simulink model "lab02_fechado"  (Simulink 10.3)
settings: Solver=VariableStepAuto  StartTime=0.0  StopTime=10.0  RelTol=1e-3
values from neighbouring files (symbols this model uses):
  c_1 = 0.2254    [lab02.mat]    (also in lab03.mat; lab04.mat; lab05.mat; lab06.mat)
  c_r = 0.0144    [lab02.mat]    (also in lab03.mat; lab04.mat; lab05.mat; lab06.mat)
  Denth = [1 1.28221624265 36.6770172992 23.5454339835 -528.584013296]    [lab03.mat]    (also in lab04.mat; lab05.mat; lab06.mat; lab07.mat)
  Denx = [1 1.28221624265 36.6770172992 23.5454339835 -528.584013296]    [lab03.mat]    (also in lab04.mat; lab05.mat; lab06.mat; lab07.mat)
  g = 9.8    [lab02.mat]    (also in lab03.mat; lab04.mat; lab05.mat; lab06.mat)
  Ja = 0.06904489    [lab02.mat]    (also in lab03.mat; lab04.mat; lab05.mat = 0.06191089; lab06.mat = 0.06932089)
  Jb = 0.04317025    [lab02.mat]    (also in lab03.mat; lab04.mat; lab05.mat = 0.03603625; lab06.mat = 0.04344625)
  k_a = 2546    [lab02.mat]    (also in lab03.mat; lab04.mat; lab05.mat; lab06.mat)
  k_f = 0.0013    [lab02.mat]    (also in lab03.mat; lab04.mat; lab05.mat; lab06.mat)
  k_hw = 2088.32    [lab02.mat]    (also in lab03.mat; lab04.mat; lab05.mat; lab06.mat)
  k_p = 2    [lab02.mat]    (also in lab03.mat = 0.256097247605; lab04.mat = 0.137612608424; lab05.mat = 0.280842058008; lab06.mat = 0.012)
  k_pf = 1    [lab02.mat]    (also in lab03.mat; lab04.mat; lab05.mat; lab06.mat)
  k_s = 32    [lab02.mat]    (also in lab03.mat; lab04.mat; lab05.mat; lab06.mat)
  k_v = 0.01    [lab02.mat]    (also in lab03.mat; lab04.mat; lab05.mat; lab06.mat)
  k_x = 50200    [lab02.mat]    (also in lab03.mat; lab04.mat; lab05.mat; lab06.mat)
  l_0 = 0.33    [lab02.mat]    (also in lab03.mat; lab04.mat; lab05.mat; lab06.mat)
  l_c = -0.0458067226891    [lab03.mat]    (also in lab04.mat; lab05.mat = -0.0295602240896; lab06.mat = -0.0463669467787; lab07.mat = -0.0295602240896)
  m_1 = 0.2376    [lab02.mat]    (also in lab03.mat; lab04.mat; lab05.mat; lab06.mat)
  m_2 = 1.785    [lab02.mat]    (also in lab03.mat; lab04.mat; lab05.mat; lab06.mat)
  Numth = [0 0 -7.64415309154 -7.25165028128 227.008182718]    [lab03.mat]    (also in lab04.mat; lab05.mat; lab06.mat; lab07.mat)
  Numx = [0 0 6.73132472896 2.24532116671 3.20735046038]    [lab03.mat]    (also in lab04.mat; lab05.mat; lab06.mat; lab07.mat)
settings Model: Creator=kisdev  LastModifiedBy=kisdev
settings SolverCC: AlgebraicLoopSolver=Auto
settings DataIOCC: SaveFormat=Dataset  SignalLoggingSaveFormat=Dataset  ReturnWorkspaceOutputs=on
settings OptimizationCC: ExpressionDepthLimit=128  LifeSpan=auto
settings DebuggingCC: UnderspecifiedInitializationDetection=Simplified  MergeDetectMultiDrivingBlocksExec=error  FcnCallInpInsideContextMsg=error  StateNameClashWarn=none  SFUnexpectedBacktrackingDiag=error  SFNoUnconditionalDefaultTransitionDiag=error  SFExecutionAtInitializationDiag=warning  SFMachineParentedDataDiag=error  ArithmeticOperatorsInVariantConditions=error
settings HardwareCC: ProdBitPerPointer=64  ProdBitPerSizeT=64  ProdBitPerPtrDiffT=64  ProdLargestAtomicFloat=Float  ProdIntDivRoundTo=Zero  ProdEndianess=LittleEndian  ProdWordSize=64  ProdHWDeviceType=Intel->x86-64 (Windows64)
settings ModelReferenceCC: PropagateSignalLabelsOutOfModel=on
settings SFSimCC: SimUseLocalCustomCode=on  CustomCodeUndefinedFunction=FilterOut
settings RTWCC: RTWUseLocalCustomCode=on
settings CodeAppCC: StateflowObjectComments=off
settings GRTTargetCC: TargetLangStandard=C99 (ISO)  CombineOutputUpdateFcns=on  GRTInterface=off
settings ConfigComp: CovMetricSettings=dwe  CovSaveCumulativeToWorkspaceVar=off  CovSaveSingleToWorkspaceVar=off  CovExternalEMLEnable=on

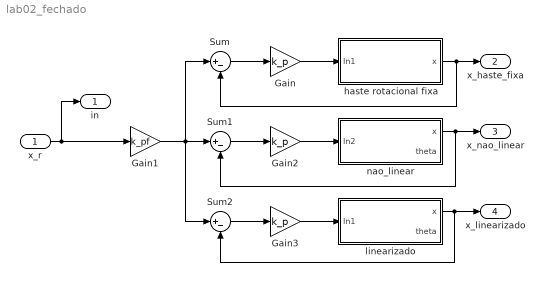
== system lab02_fechado ==
  x_r : Inport
  Gain : Gain  Gain=k_p
  Gain1 : Gain  Gain=k_pf
  Gain2 : Gain  Gain=k_p
  Gain3 : Gain  Gain=k_p
  Sum : Sum  Inputs=|+-
  Sum1 : Sum  Inputs=|+-
  Sum2 : Sum  Inputs=|+-
  haste rotacional fixa : Subsystem
  linearizado : Subsystem
  nao_linear : Subsystem
  in : Outport
  x_haste_fixa : Outport  Port=2
  x_nao_linear : Outport  Port=3
  x_linearizado : Outport  Port=4
  wires:
  x_r/1 -> in/1, Gain1/1
  Gain1/1 -> Sum2/1, Sum1/1, Sum/1
  Sum/1 -> Gain/1
  Sum1/1 -> Gain2/1
  Sum2/1 -> Gain3/1
  nao_linear/1(x) -> Sum1/2, x_nao_linear/1
  Gain2/1 -> nao_linear/1(In2)
  Gain/1 -> haste rotacional fixa/1(In1)
  haste rotacional fixa/1(x) -> Sum/2, x_haste_fixa/1
  Gain3/1 -> linearizado/1(In1)
  linearizado/1(x) -> Sum2/2, x_linearizado/1

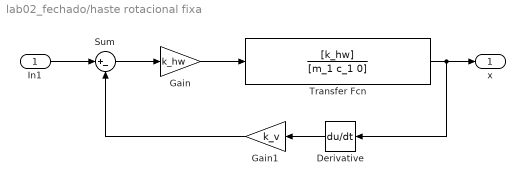
== system lab02_fechado/haste rotacional fixa ==
  In1 : Inport
  Derivative : Derivative
  Gain : Gain  Gain=k_hw
  Gain1 : Gain  Gain=k_v
  Sum : Sum  Inputs=|+-
  Transfer Fcn : TransferFcn  Numerator=[k_hw]  Denominator=[m_1 c_1 0]
  x : Outport
  wires:
  Transfer Fcn/1 -> Derivative/1, x/1
  Derivative/1 -> Gain1/1
  Gain1/1 -> Sum/2
  Gain/1 -> Transfer Fcn/1
  In1/1 -> Sum/1
  Sum/1 -> Gain/1

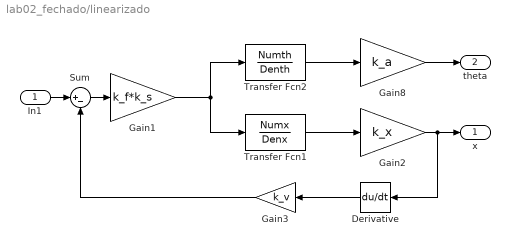
== system lab02_fechado/linearizado ==
  In1 : Inport
  Derivative : Derivative
  Gain1 : Gain  Gain=k_f*k_s
  Gain2 : Gain  Gain=k_x
  Gain3 : Gain  Gain=k_v
  Gain8 : Gain  Gain=k_a
  Sum : Sum  Inputs=|+-
  Transfer Fcn1 : TransferFcn  Numerator=Numx  Denominator=Denx
  Transfer Fcn2 : TransferFcn  Numerator=Numth  Denominator=Denth
  x : Outport
  theta : Outport  Port=2
  wires:
  Sum/1 -> Gain1/1
  In1/1 -> Sum/1
  Gain2/1 -> x/1, Derivative/1
  Transfer Fcn2/1 -> Gain8/1
  Gain1/1 -> Transfer Fcn1/1, Transfer Fcn2/1
  Transfer Fcn1/1 -> Gain2/1
  Gain8/1 -> theta/1
  Gain3/1 -> Sum/2
  Derivative/1 -> Gain3/1

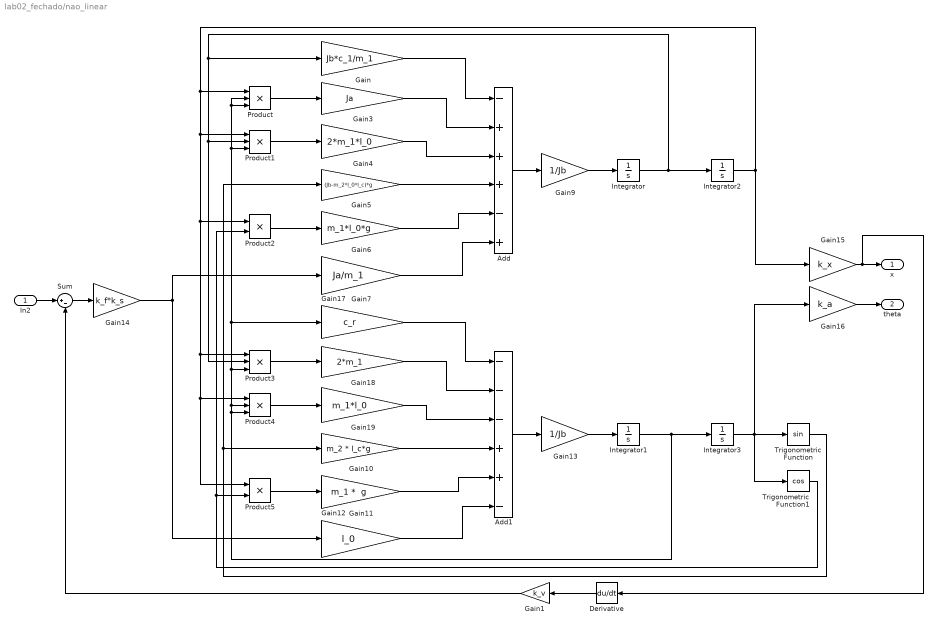
== system lab02_fechado/nao_linear ==
  In2 : Inport
  Add : Sum  Inputs=-+++-+
  Add1 : Sum  Inputs=---++-
  Derivative : Derivative
  Gain : Gain  Gain=Jb*c_1/m_1
  Gain1 : Gain  Gain=k_v
  Gain10 : Gain  Gain=m_2 * l_c*g
  Gain11 : Gain  Gain="m_1 *  g"
  Gain12 : Gain  Gain=l_0
  Gain13 : Gain  Gain=1/Jb
  Gain14 : Gain  Gain=k_f*k_s
  Gain15 : Gain  Gain=k_x
  Gain16 : Gain  Gain=k_a
  Gain17 : Gain  Gain=c_r
  Gain18 : Gain  Gain=2*m_1
  Gain19 : Gain  Gain=m_1*l_0
  Gain3 : Gain  Gain=Ja
  Gain4 : Gain  Gain=2*m_1*l_0
  Gain5 : Gain  Gain=(Jb-m_2*l_0*l_c)*g
  Gain6 : Gain  Gain=m_1*l_0*g
  Gain7 : Gain  Gain=Ja/m_1
  Gain9 : Gain  Gain=1/Jb
  Integrator{,1..3} (4 alike) : Integrator
  Product{,1,3..4} (4 alike) : Product  Inputs=3
  Product2 : Product
  Product5 : Product
  Sum : Sum  Inputs=|+-
  Trigonometric Function : Trigonometry
  Trigonometric Function1 : Trigonometry  Operator=cos
  x : Outport
  theta : Outport  Port=2
  wires:
  Gain9/1 -> Integrator/1
  Integrator3/1 -> Gain16/1, Trigonometric Function1/1, Trigonometric Function/1
  Integrator2/1 -> Gain15/1, Product5/1, Product4/1, Product3/1, Product2/1, Product1/1, Product/1
  Gain/1 -> Add/1
  Gain4/1 -> Add/3
  Add/1 -> Gain9/1
  Product4/1 -> Gain19/1
  Gain11/1 -> Add1/5
  Sum/1 -> Gain14/1
  Gain13/1 -> Integrator1/1
  In2/1 -> Sum/1
  Product2/1 -> Gain6/1
  Gain17/1 -> Add1/1
  Product/1 -> Gain3/1
  Gain12/1 -> Add1/6
  Integrator1/1 -> Product4/3, Product4/2, Product3/3, Gain17/1, Product1/3, Product/3, Product/2, Integrator3/1
  Gain5/1 -> Add/4
  Gain10/1 -> Add1/4
  Gain14/1 -> Gain12/1, Gain7/1
  Integrator/1 -> Gain/1, Product3/2, Product1/2, Integrator2/1
  Gain15/1 -> x/1, Derivative/1
  Gain6/1 -> Add/5
  Product1/1 -> Gain4/1
  Product3/1 -> Gain18/1
  Gain18/1 -> Add1/2
  Trigonometric Function1/1 -> Product5/2, Product2/2
  Gain16/1 -> theta/1
  Gain3/1 -> Add/2
  Trigonometric Function/1 -> Gain10/1, Gain5/1
  Gain19/1 -> Add1/3
  Add1/1 -> Gain13/1
  Gain7/1 -> Add/6
  Product5/1 -> Gain11/1
  Derivative/1 -> Gain1/1
  Gain1/1 -> Sum/2
